simulink library "adcs_mpc_main"  (R2016b)
settings: Solver=VariableStepAuto  StartTime=0.0  StopTime=10.0  RelTol=1e-3
undefined symbols (not defined in the file): command, status
libraries: mpclib x1, linearization x1, bus_stubs_fsw x1
settings Model: Creator=bijan  LastModifiedBy=bijan

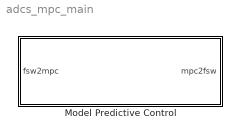
== system adcs_mpc_main ==
  Model Predictive Control : Subsystem

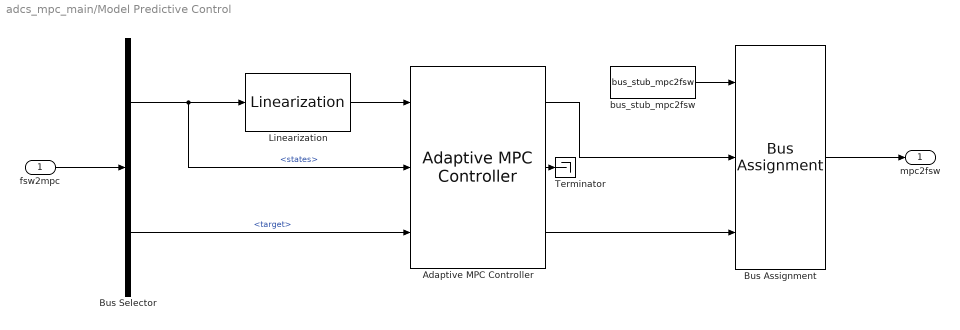
== system adcs_mpc_main/Model Predictive Control ==
  fsw2mpc : Inport  OutDataTypeStr=Bus: fsw2mpc
  Adaptive MPC Controller : mpclib/Adaptive MPC Controller  SCDEnableBlockLinearizationSpecification=on  mpcobj=fsw_params.control.mpc.MPCobject  md_inport=off  mv_inport=off  cost_outport=off  return_sequence=on  return_qpstatus=on  return_state=off  state_inport=on  isltv_plant=off  lims_inport=off  cc_inport=off  ywt_inport=off  uwt_inport=off  duwt_inport=off  rhoeps_inport=off  uref_inport=off  BlockDataType=double  SampleTimeInherited=off  switch_inport=off
  Bus Assignment : BusAssignment  AssignedSignals=command,status
  Bus Selector : BusSelector  OutputSignals=states,target
  Linearization : linearization/Linearization
  Terminator : Terminator
  bus_stub_mpc2fsw : bus_stubs_fsw/bus_stub_mpc2fsw
  mpc2fsw : Outport
  wires:
  fsw2mpc/1 -> Bus Selector/1
  Bus Selector/1 -> Adaptive MPC Controller/2, Linearization/1  "<states>"
  Adaptive MPC Controller/2 -> Terminator/1
  Bus Selector/2 -> Adaptive MPC Controller/3  "<target>"
  Adaptive MPC Controller/3 -> Bus Assignment/3
  Adaptive MPC Controller/1 -> Bus Assignment/2
  bus_stub_mpc2fsw/1 -> Bus Assignment/1
  Bus Assignment/1 -> mpc2fsw/1
  Linearization/1 -> Adaptive MPC Controller/1
